simulink model "Bicycel_Model"  (R2025b)
settings: Solver=FixedStepAuto  StartTime=0.0  StopTime=15  RelTol=1e-3
libraries: autolibshared x2
settings Model: Creator=thoma  LastModifiedBy=thoma

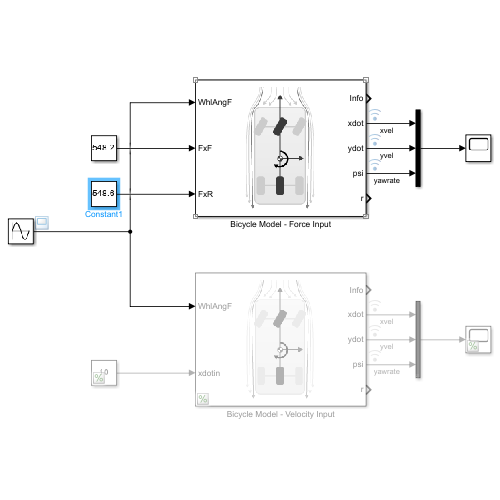
[thumbnail: Simulink's stored preview of the top-level diagram]
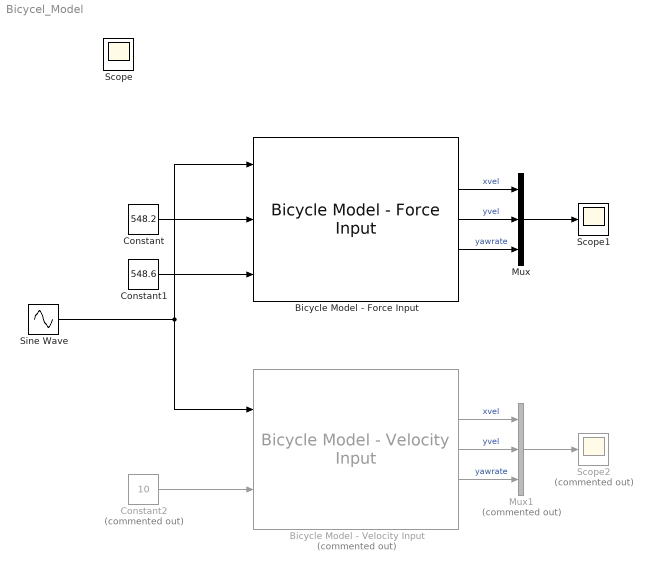
== system Bicycel_Model ==
  Bicycle Model - Force Input : autolibshared/Bicycle Model - Force Input  trackMode=Single (bicycle)  inputMode=External longitudinal forces  frontSteerMode=on  rearSteerMode=off  windMode=off  muMode=off  extFMode=off  extMMode=off  aMode=2  NF=2  NR=2  m=270  a=0.68  b=0.86  h=0.037  X_o=0  xdot_o=0  CalphaMode=off  sigmaMode=on  w=[1.4,1.4]  Cy_f=12e3  Cy_r=11e3  sigma_f=.1  sigma_r=.1  alpha_f_brk=[-.1 .1]  Cy_f_data=[-9e3 9e3]  alpha_r_brk=[-.1 .1]  Cy_r_data=[-9e3 9e3]  Y_o=0  ydot_o=0  Izz=4000  psi_o=0  r_o=0  Af=0.810  Cd=1.400  Cl=4.230  Cpm=.1  beta_w=[0 0.01:0.01:0.3]  Cs=[0 0.01:0.01:0.3]  Cym=[0 1e-6:0.01:0.3]  Pabs=101325  Tair=273  g=9.81  mu=1  xdot_tol=.01  Fznom=5000  Fxtire_sat=1e6  Fytire_sat=1e6  longOff=0  latOff=0  vertOff=0
      settings: LibrarySourceBlock=vehdynlibeom/Bicycle Model - Force Input
  Bicycle Model - Velocity Input : autolibshared/Bicycle Model - Velocity Input  Commented=on  trackMode=Single (bicycle)  inputMode=External longitudinal velocity  frontSteerMode=on  rearSteerMode=off  windMode=off  muMode=off  extFMode=off  extMMode=off  aMode=2  NF=2  NR=2  m=270  a=0.68  b=0.86  h=0.35  X_o=0  xdot_o=0  CalphaMode=off  sigmaMode=on  w=[1.4,1.4]  Cy_f=12e3  Cy_r=11e3  sigma_f=.1  sigma_r=.1  alpha_f_brk=[-.1 .1]  Cy_f_data=[-9e3 9e3]  alpha_r_brk=[-.1 .1]  Cy_r_data=[-9e3 9e3]  Y_o=0  ydot_o=0  Izz=4000  psi_o=0  r_o=0  Af=0.810  Cd=1.4  Cl=4.230  Cpm=.1  beta_w=[0 0.01:0.01:0.3]  Cs=[0 0.01:0.01:0.3]  Cym=[0 1e-6:0.01:0.3]  Pabs=101325  Tair=273  g=9.81  mu=1  xdot_tol=.01  Fznom=5000  Fxtire_sat=1e6  Fytire_sat=1e6  longOff=0  latOff=0  vertOff=0
      settings: LibrarySourceBlock=vehdynlibeom/Bicycle Model - Velocity Input
  Constant : Constant  Value=548.2
  Constant1 : Constant  Value=548.6
  Constant2 : Constant  Commented=on  Value=10
  Mux : Mux  Inputs=3
  Mux1 : Mux  Commented=on  Inputs=3
  Scope1 : Scope
      settings: ActiveDisplayYMinimum=-7.7683065504283624  ActiveDisplayYMaximum=5.5907511391320082
  Scope2 : Scope  Commented=on
      settings: ActiveDisplayYMinimum=-9.32605017271369  ActiveDisplayYMaximum=4.1927070072132535  DataLoggingVariableName=ScopeData2
  Sine Wave : Sin  Amplitude=3  Frequency=0.5  SampleTime=0
  Scope : Scope
  wires:
  Sine Wave/1 -> Bicycle Model - Velocity Input/1, Bicycle Model - Force Input/1
  Bicycle Model - Force Input/3 -> Mux/2  "yvel"
  Bicycle Model - Force Input/4 -> Mux/3  "yawrate"
  Constant/1 -> Bicycle Model - Force Input/2
  Constant1/1 -> Bicycle Model - Force Input/3
  Constant2/1 -> Bicycle Model - Velocity Input/2
  Bicycle Model - Force Input/2 -> Mux/1  "xvel"
  Mux/1 -> Scope1/1
  Bicycle Model - Velocity Input/2 -> Mux1/1  "xvel"
  Mux1/1 -> Scope2/1
  Bicycle Model - Velocity Input/4 -> Mux1/3  "yawrate"
  Bicycle Model - Velocity Input/3 -> Mux1/2  "yvel"
